simulink model "statefdbk"  (R2021b)
settings: Solver=VariableStepAuto  StartTime=0.0  StopTime=2  RelTol=1e-3
values from neighbouring files (symbols this model uses):
  C = diag([1,1,1,1,1])    [inv_pendulum.m]
  D = [0 0 0 0 0]'    [inv_pendulum.m]
  K = lqr(A, B, Qr, Rr)    [inv_pendulum.m]
  x0 = [0.1 0 0 0 0]'    [inv_pendulum.m]
undefined symbols (not defined in the file or in its folder): A, B
settings Model: Creator=freed  LastModifiedBy=freed

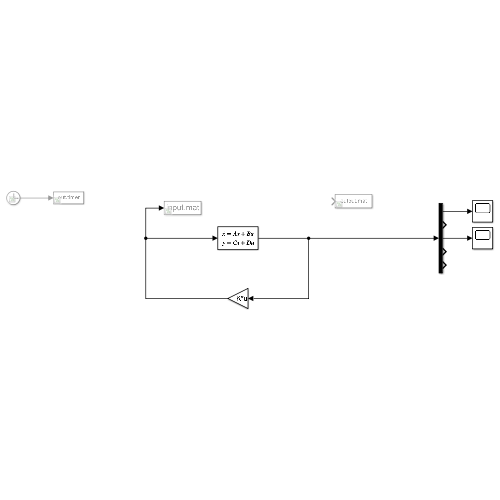
[thumbnail: Simulink's stored preview of the top-level diagram]
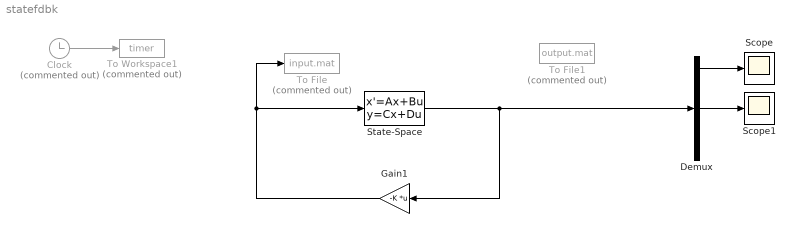
== system statefdbk ==
  Clock : Clock  Commented=on
  Demux : Demux  Outputs=5
  Gain1 : Gain  Gain=-K  Multiplication=Matrix(K*u)
  Scope : Scope
  Scope1 : Scope
  State-Space : StateSpace  A=A  B=B  C=C  D=D  InitialCondition=x0  ParameterTunability=Unconstrained
  To File : ToFile  Commented=on  Filename=input.mat  MatrixName=u
  To File1 : ToFile  Commented=on  Filename=output.mat  MatrixName=y
  To Workspace1 : ToWorkspace  Commented=on  VariableName=timer  SaveFormat=Timeseries  SampleTime=-1
  wires:
  State-Space/1 -> Demux/1, Gain1/1
  Gain1/1 -> To File/1, State-Space/1
  Clock/1 -> To Workspace1/1
  Demux/1 -> Scope/1
  Demux/3 -> Scope1/1
